simulink subsystem "DrivingPatternBasic_refsub"  (R2020b)
settings: Solver=VariableStepAuto  StartTime=0.0  StopTime=10.0  RelTol=1e-3
undefined symbols (not defined in the file or in its folder): drivingPattern
libraries: autolibshared x1
settings Model: Creator=isaacito  LastModifiedBy=isaacito

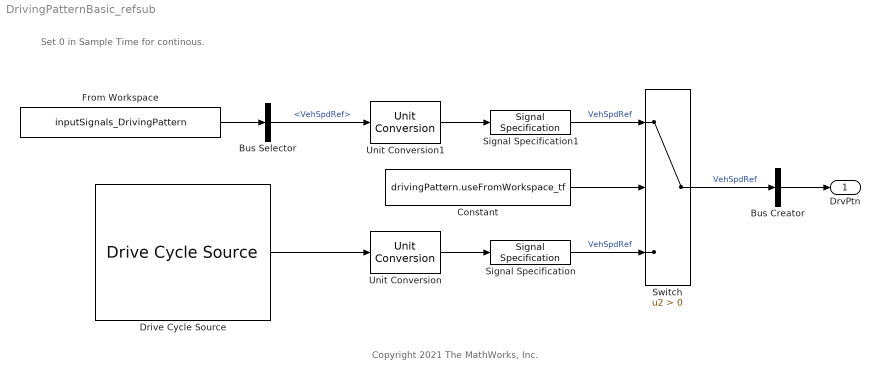
== system DrivingPatternBasic_refsub ==
  note: Copyright 2021 The MathWorks, Inc.
  note: Set 0 in Sample Time for continous.
  Bus Creator : BusCreator  Inputs=1
  Bus Selector : BusSelector  OutputSignals=VehSpdRef
  Constant : Constant  Value=drivingPattern.useFromWorkspace_tf
  Drive Cycle Source : autolibshared/Drive Cycle Source  cycleVar=FTP75  fileVar=cycleFTP75.mat  tfinal="2474  seconds"  cycleRepeat=off  outAccPort=off  outGearPort=off  gearList=No gear data  t_wot1=5  xdot_woto=0  xdot_wot1=30  t_wot2=20  xdot_wot2=0  t_wotend=30  srcUnit=m/s  outUnit=mph  srcAccUnit=m/s/s  outAccUnit=m/s^2  dt=0  aMode=1  faultOption=off  velBnd=2  velBndUnit=mph  inUnit=m/s  timeBnd=1  failOption=off  stopSim=off  maxFaultCnt=10  maxFaultTime=2  maxTotFaultTime=15  traceOption=off  dtTrace=1  traceWindow=10  lastDCname=FTP75 Velocity  lastOutUnit=mph  lastDT=0  lastTB=1  lastSB=2  forceCalcBound=off
      settings: SourceProductBaseCode=PW,MT,UV,VE,VP
  From Workspace : FromWorkspace  VariableName=inputSignals_DrivingPattern  OutDataTypeStr=Bus: inputBus_DrivingPattern  OutputAfterFinalValue=Holding final value
      settings: AttributesFormatString=|
      | %<OutDataTypeStr>
      | Sample Time: %<SampleTime>
  Signal Specification : SignalSpecification  Unit=m/s
  Signal Specification1 : SignalSpecification  Unit=m/s
  Switch : Switch  Criteria=u2 > Threshold
  Unit Conversion : UnitConversion
  Unit Conversion1 : UnitConversion
  DrvPtn : Outport
  wires:
  Bus Selector/1 -> Unit Conversion1/1  "<VehSpdRef>"
  Signal Specification1/1 -> Switch/1  "VehSpdRef"
  Unit Conversion1/1 -> Signal Specification1/1
  Switch/1 -> Bus Creator/1  "VehSpdRef"
  Signal Specification/1 -> Switch/3  "VehSpdRef"
  Drive Cycle Source/1 -> Unit Conversion/1
  Unit Conversion/1 -> Signal Specification/1
  Bus Creator/1 -> DrvPtn/1
  From Workspace/1 -> Bus Selector/1
  Constant/1 -> Switch/2
